simulink model "operationalSpaceInverseDynamicsControl_compliance"  (R2021a)
settings: Solver=VariableStepAuto  StartTime=0.0  StopTime=5  RelTol=1e-3
values from neighbouring files (symbols this model uses):
  K = diag([0 10 0 0 0 10])    [assignment12_main.m]
  Kd = diag([10, 10, 10, 10, 10, 10])    [assignment12_main.m]
  Kp = diag([30, 30, 30, 30, 30, 30])    [assignment12_main.m]
  M_d = 0.1*diag([10 10 10 10 10 10])    [assignment12_main.m]
  x_d_const = [0.00001 -0.3 0.5 pi/2 -pi/2 0].'    [assignment12_main.m]
libraries: vrlib x1, robotcorelib x1
settings Model: Creator=fabio  LastModifiedBy=fabio

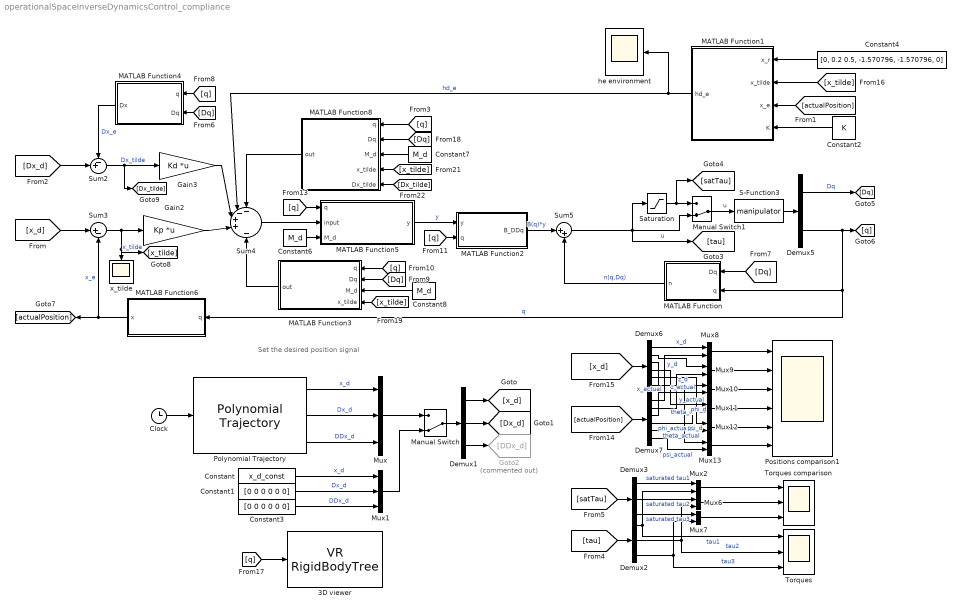
== system operationalSpaceInverseDynamicsControl_compliance ==
  note: Set the desired position signal
  3D viewer : vrlib/VR RigidBodyTree  RBT=robot  useRBT=off  Ts=-1  ForceViewerOpen=on
      settings: SourceProductBaseCode=SL
  Clock : Clock
  Constant : Constant  Value=x_d_const
  Constant1 : Constant  Value=[0 0 0 0 0 0]
  Constant2 : Constant  Value=K  VectorParams1D=off
  Constant3 : Constant  Value=[0 0 0 0 0 0]
  Constant4 : Constant  Value=[0, 0.2 0.5, -1.570796, -1.570796, 0]
  Constant6 : Constant  Value=M_d  VectorParams1D=off
  Constant7 : Constant  Value=M_d  VectorParams1D=off
  Constant8 : Constant  Value=M_d  VectorParams1D=off
  Demux1 : Demux  Outputs=3
  Demux2 : Demux  Outputs=3
  Demux3 : Demux  Outputs=3
  Demux5 : Demux  Outputs=[3 3]
  Demux6 : Demux  Outputs=6
  Demux7 : Demux  Outputs=6
  Gain2 : Gain  Gain=Kp  Multiplication=Matrix(K*u) (u vector)
  Gain3 : Gain  Gain=Kd  Multiplication=Matrix(K*u) (u vector)
  Goto2 : Goto  Commented=on  GotoTag=DDx_d
  MATLAB Function : MATLAB Function  TreatAsAtomicUnit=on
  MATLAB Function1 : MATLAB Function  TreatAsAtomicUnit=on
  MATLAB Function2 : MATLAB Function  TreatAsAtomicUnit=on
  MATLAB Function3 : MATLAB Function  TreatAsAtomicUnit=on
  MATLAB Function4 : MATLAB Function  TreatAsAtomicUnit=on
  MATLAB Function5 : MATLAB Function  TreatAsAtomicUnit=on
  MATLAB Function6 : MATLAB Function  TreatAsAtomicUnit=on
  MATLAB Function8 : MATLAB Function  TreatAsAtomicUnit=on
  Manual Switch : ManualSwitch  CurrentSetting=0
  Manual Switch1 : ManualSwitch  CurrentSetting=0
  Mux : Mux  Inputs=3
  Mux1 : Mux  Inputs=3
  Mux{2,6..13} (9 alike) : Mux  Inputs=2
  Polynomial Trajectory : robotcorelib/Polynomial Trajectory  WaypointSource=Internal  Waypoints=x_d  TimePoints=[ 0, 10, 20]  TimeInterval=[ 1, 4 ]  Method=Cubic Polynomial  ParameterSource=Internal  VelocityBoundaryCondition=zeros( 6, 3)  AccelerationBoundaryCondition=zeros( 2, 5 )  SimulateUsing=Interpreted execution
  Positions comparison1 : Scope  NumInputPorts=6
  S-Function3 : S-Function  FunctionName=manipulator  Parameters=myRobot  SFunctionDeploymentMode=off  EnableBusSupport=off
  Saturation : Saturate  UpperLimit=20  LowerLimit=-20
  Sum2 : Sum  Inputs=-+|
  Sum3 : Sum  Inputs=|+-
  Sum4 : Sum  Inputs=--++|-
  Sum5 : Sum  Inputs=|++
  Torques : Scope  NumInputPorts=3
  Torques comparison : Scope  NumInputPorts=3
  he environment : Scope
  x_tilde : Scope
  wires:
  Manual Switch1/1 -> S-Function3/1  "u"
  Sum3/1 -> Gain2/1, [x_tilde], x_tilde/1  "x_tilde"
  S-Function3/1 -> Demux5/1
  Demux5/1 -> [Dq]  "Dq"
  Demux5/2 -> MATLAB Function6/1(q), MATLAB Function/2(q), [q]  "q"
  Gain2/1 -> Sum4/4
  Sum2/1 -> [Dx_tilde], Gain3/1  "Dx_tilde"
  Gain3/1 -> Sum4/3
  Sum4/1 -> MATLAB Function5/2(input)
  MATLAB Function2/1(B_DDq) -> Sum5/1  "B(q)*y"
  MATLAB Function/1(n) -> Sum5/2  "n(q,Dq)"
  Clock/1 -> Polynomial Trajectory/1
  Polynomial Trajectory/2 -> Mux/2  "Dx_d"
  [x_d] -> Sum3/1
  [Dx_d] -> Sum2/2
  Polynomial Trajectory/1 -> Mux/1  "x_d"
  Polynomial Trajectory/3 -> Mux/3  "DDx_d"
  Mux/1 -> Manual Switch/1
  Manual Switch/1 -> Demux1/1
  Demux1/1 -> [x_d]
  Demux1/2 -> [Dx_d]
  Demux1/3 -> Goto2/1
  Constant/1 -> Mux1/1  "x_d"
  Constant1/1 -> Mux1/2  "Dx_d"
  Mux1/1 -> Manual Switch/2
  Constant3/1 -> Mux1/3  "DDx_d"
  Demux2/1 -> Torques/1, Mux2/2  "tau1"
  [tau] -> Demux2/1
  Saturation/1 -> [satTau], Manual Switch1/1
  [satTau] -> Demux3/1
  Demux3/1 -> Mux2/1  "saturated tau1"
  Mux2/1 -> Torques comparison/1
  Mux6/1 -> Torques comparison/2
  Mux7/1 -> Torques comparison/3
  Demux2/2 -> Torques/2, Mux6/2  "tau2"
  Demux3/2 -> Mux6/1  "saturated tau2"
  Demux3/3 -> Mux7/1  "saturated tau3"
  Demux2/3 -> Torques/3, Mux7/2  "tau3"
  MATLAB Function6/1(x) -> Sum3/2, [actualPosition]  "x_e"
  [Dq] -> MATLAB Function/1(Dq)
  [Dq] -> MATLAB Function4/2(Dq)
  [q] -> MATLAB Function4/1(q)
  MATLAB Function4/1(Dx) -> Sum2/1  "Dx_e"
  [Dq] -> MATLAB Function3/2(Dq)
  [q] -> MATLAB Function3/1(q)
  MATLAB Function3/1(out) -> Sum4/5
  [q] -> MATLAB Function2/2(q)
  [q] -> MATLAB Function5/1(q)
  MATLAB Function5/1(y) -> MATLAB Function2/1(y)  "y"
  Demux6/2 -> Mux9/1  "y_d"
  Demux7/2 -> Mux9/2  "y_actual"
  [x_d] -> Demux6/1
  Demux6/5 -> Mux12/1  "theta_d"
  Demux7/1 -> Mux8/2  "x_actual"
  Demux6/4 -> Mux11/1  "phi_d"
  Demux7/4 -> Mux11/2  "phi_actual"
  Demux7/5 -> Mux12/2  "theta_actual"
  Demux7/6 -> Mux13/2  "psi_actual"
  Mux13/1 -> Positions comparison1/6
  Mux9/1 -> Positions comparison1/2
  Mux8/1 -> Positions comparison1/1
  Mux10/1 -> Positions comparison1/3
  [actualPosition] -> Demux7/1
  Demux6/1 -> Mux8/1  "x_d"
  Mux11/1 -> Positions comparison1/4
  Demux7/3 -> Mux10/2  "z_actual"
  Demux6/6 -> Mux13/1  "psi_d"
  Mux12/1 -> Positions comparison1/5
  Demux6/3 -> Mux10/1  "z_d"
  Constant4/1 -> MATLAB Function1/1(x_r)
  [actualPosition] -> MATLAB Function1/3(x_e)
  [x_tilde] -> MATLAB Function1/2(x_tilde)
  Constant2/1 -> MATLAB Function1/4(K)
  Sum5/1 -> Saturation/1, Manual Switch1/2, [tau]  "u"
  [q] -> 3D viewer/1
  Constant6/1 -> MATLAB Function5/3(M_d)
  Constant8/1 -> MATLAB Function3/3(M_d)
  MATLAB Function1/1(hd_e) -> he environment/1, Sum4/2  "hd_e"
  MATLAB Function8/1(out) -> Sum4/1
  Constant7/1 -> MATLAB Function8/3(M_d)
  [Dq] -> MATLAB Function8/2(Dq)
  [q] -> MATLAB Function8/1(q)
  [x_tilde] -> MATLAB Function3/4(x_tilde)
  [x_tilde] -> MATLAB Function8/4(x_tilde)
  [Dx_tilde] -> MATLAB Function8/5(Dx_tilde)

== matlab function operationalSpaceInverseDynamicsControl_compliance/MATLAB Function1 ==
  data: x_r input; x_tilde input; x_e input; K input; hd_e output
function hd_e  = environment(x_r, x_tilde, x_e, K)
    
    phi_d_e = -x_tilde(4:6);
    
    %Compute T(phi_d_e) function of the euler angles of x_d
    T = [0, -sin(phi_d_e(1)), cos(phi_d_e(1))*sin(phi_d_e(2));
         0,  cos(phi_d_e(1)), sin(phi_d_e(1))*sin(phi_d_e(2));
         1,     0           , cos(phi_d_e(2))                ];

    Ta = [1 0 0   0 0 0 ;
          0 1 0   0 0 0 ;
          0 0 1   0 0 0 ;
          0 0 0 , T(1,:);
          0 0 0 , T(2,:);
          0 0 0 , T(3,:)];    
   
    
    y_plane = x_r(2);
    %contact with the plane
    if size(x_e,1) > 1 && x_e(2) > y_plane 
        dx_re = x_e - x_r;
        h_e = K * dx_re;
    else %no contact with the plane
        h_e = [0 0 0 0 0 0].';
    end
    
    hd_e = Ta.'*h_e;
end

== matlab function operationalSpaceInverseDynamicsControl_compliance/MATLAB Function ==
  data: Dq input; n output; q input
function n = n_q_Dq(Dq, q)
    
    %To get the "perfect" matrices use the following code
    C = get_C_matrix(q,Dq);
    G = get_G_matrix(q);
    
    
    %To get the "wrongly estimated" matrices use the following code   
%     theta2 = q(2);   d3 = q(3); 
%     Dtheta2 = Dq(2); Dd3 = Dq(3); 
%     
%     m_Link4 = 0.16;  %0.2kg is the correct value
% 
%     C = [0,                         0,                        0;
%          0,            m_Link4*Dd3*d3,       m_Link4*Dtheta2*d3;
%          0,       -m_Link4*Dtheta2*d3,                        0];
%    
%     G = [           0                           ;
%          (981*m_Link4*sin(theta2)*d3)/100 ;
%           -(981*m_Link4*cos(theta2))/100    ];


    
    n = C*Dq + G; %F = friction is neglected

end

== matlab function operationalSpaceInverseDynamicsControl_compliance/MATLAB Function2 ==
  data: y input; B_DDq output; q input
function B_DDq = B_q(y,q)
    B_DDq = get_B_matrix(q)*y;
end

== matlab function operationalSpaceInverseDynamicsControl_compliance/MATLAB Function3 ==
  data: q input; out output; Dq input; M_d input; x_tilde input
function out = DJad_x_Dq(q, Dq, M_d, x_tilde)
    %Compute the numerical derivative of the analytical jacobian
    theta2 = q(2);
    d3 = q(3);
    Dtheta2 = Dq(2);
    Dd3 = Dq(3);
     
    Rd = eul2rotm(-x_tilde(4:6).', 'ZYZ');
    phi_d_e = -x_tilde(4:6);
    
    %Compute T(phi_d_e) function of the euler angles of x_d
    T = [0, -sin(phi_d_e(1)), cos(phi_d_e(1))*sin(phi_d_e(2));
         0,  cos(phi_d_e(1)), sin(phi_d_e(1))*sin(phi_d_e(2));
         1,     0           , cos(phi_d_e(2))                ];

    Ta = [1 0 0   0 0 0 ;
          0 1 0   0 0 0 ;
          0 0 1   0 0 0 ;
          0 0 0 , T(1,:);
          0 0 0 , T(2,:);
          0 0 0 , T(3,:)];    
      
    %Geometric jacobian w.r.t. to frame 0
    L4 = 0.4;
    DJg = [0, cos(theta2)*Dd3 + sin(theta2)*(L4/2 - d3)*Dtheta2, cos(theta2)*Dtheta2;
           0, sin(theta2)*Dd3 - cos(theta2)*(L4/2 - d3)*Dtheta2, sin(theta2)*Dtheta2;
           0,                        0,            0;
           0,                        0,            0;
           0,                        0,            0;
           0,                        0,            0];

       
    DJad = pinv(Ta)*[Rd.'        zeros(3,3);
                     zeros(3,3)  Rd.'      ] * DJg;
           
    out = M_d * DJad * Dq;
      
end

== matlab function operationalSpaceInverseDynamicsControl_compliance/MATLAB Function4 ==
  data: q input; Dx output; Dq input
function Dx = Ja_x_Dq(q, Dq)
    %Compute the numerical analytical jacobian
    theta2 = q(2);
    d3 = q(3);
    
    %Manually pasted (not possible otherwise) Ja from ∑0 to ∑ee 
    L4 = 0.4;
    Ja = [0, -cos(theta2)*(L4/2 - d3),  sin(theta2);
          0, -sin(theta2)*(L4/2 - d3), -cos(theta2);
          1,                        0,            0;
          0,                        1,            0;
          0,                        0,            0;
          0,                        0,           0];
 
    Dx = Ja * Dq;
      
end

== matlab function operationalSpaceInverseDynamicsControl_compliance/MATLAB Function5 ==
  data: q input; y output; input input; M_d input
function y = invJa_x_invMd(q, input, M_d)
    %Compute the numerical analytical jacobian
    theta2 = q(2);
    d3 = q(3);
   
    %Manually pasted (not possible otherwise) Ja from ∑0 to ∑ee 
    L4 = 0.4;
    Ja = [0, -cos(theta2)*(L4/2 - d3),  sin(theta2);
          0, -sin(theta2)*(L4/2 - d3), -cos(theta2);
          1,                        0,            0;
          0,                        1,            0;
          0,                        0,            0;
          0,                        0,           0];
    
    y = pinv(Ja) * inv(M_d) * input;
 
end

== matlab function operationalSpaceInverseDynamicsControl_compliance/MATLAB Function6 ==
  data: q input; x output
function x = k(q) 
    %Compute the direct kinematics from the copied and pasted last
    %transformation matrix
    d1 = q(1);
    theta2 = q(2);
    d3 = q(3);
    
    %get rotation matrix from ∑0 to ∑ee    
    R0_to_ee = [ 0, cos(theta2), -sin(theta2);
                 0, sin(theta2),  cos(theta2);  
                 1,      0,       0         ];
             
    %get translation vector from ∑0 to ∑ee 
    L2 = 0.4; L3 = 0.3; L4 = 0.4;
    p0_to_ee = [ -sin(theta2)*(L4/2 - d3);
                 cos(theta2)*(L4/2 - d3) ;
                 L2/2 + L3 + d1         ];
                 
    eulerAngles = rotm2eul(R0_to_ee, 'ZYZ');
    
%     x = [ 0.4/2 + 0.3 + d1;
%           sin(theta2)*(0.4/2 - d3);
%           0.4 + cos(theta2)*d3 - (0.4*cos(theta2))/2;
%           eulerAngles.'];
    x = [ p0_to_ee;
          eulerAngles.' ];
    
end

== matlab function operationalSpaceInverseDynamicsControl_compliance/MATLAB Function8 ==
  data: q input; out output; Dq input; M_d input; x_tilde input; Dx_tilde input
function out = Md_x_b(q, Dq, M_d, x_tilde, Dx_tilde)
    
    theta2 = q(2);
    d3 = q(3);
    
    Rd = eul2rotm(-x_tilde(4:6).', 'ZYZ');
    phi_d_e = -x_tilde(4:6);
    
    %Compute T(phi_d_e) function of the euler angles of x_d
    T = [0, -sin(phi_d_e(1)), cos(phi_d_e(1))*sin(phi_d_e(2));
         0,  cos(phi_d_e(1)), sin(phi_d_e(1))*sin(phi_d_e(2));
         1,     0           , cos(phi_d_e(2))                ];

    Ta = [1 0 0   0 0 0 ;
          0 1 0   0 0 0 ;
          0 0 1   0 0 0 ;
          0 0 0 , T(1,:);
          0 0 0 , T(2,:);
          0 0 0 , T(3,:)];    
      
    %Geometric jacobian w.r.t. to frame 0
    L4 = 0.4;
    Jg = [0, -cos(theta2)*(L4/2 - d3),  sin(theta2);
          0, -sin(theta2)*(L4/2 - d3), -cos(theta2);
          1,                        0,            0;
          0,                        0,            0;
          0,                        0,            0;
          0,                        1,            0];

    Jad = pinv(Ta)*[Rd.'        zeros(3,3);
                     zeros(3,3)  Rd.'      ] * Jg;                 

    %According to slide 29: 
    out = M_d * (Dx_tilde + Jad*Dq);
      
end
